simulink model "Lab1_Simulation"  (R2025b)
settings: Solver=VariableStepAuto  StartTime=0.0  StopTime=2  RelTol=1e-3
values from neighbouring files (symbols this model uses):
  a0 = K/a4    (= 224637.681159)    [Lab1matlab.m]
  a1 = (K*Tau1+K*Tau2+G)/a4    (= 24764.4927536)    [Lab1matlab.m]
  a2 = (Tau1*Tau2*K+G*Tau1+G*Tau2+J)/a4    (= 1527.89855072)    [Lab1matlab.m]
  a3 = (Tau1*Tau2*G+J*Tau1+J*Tau2)/a4    (= 60.8695652174)    [Lab1matlab.m]
  b0 = 1/a4    (= 226449.275362)    [Lab1matlab.m]
settings Model: Creator=peterbarkley  LastModifiedBy=peterbarkley

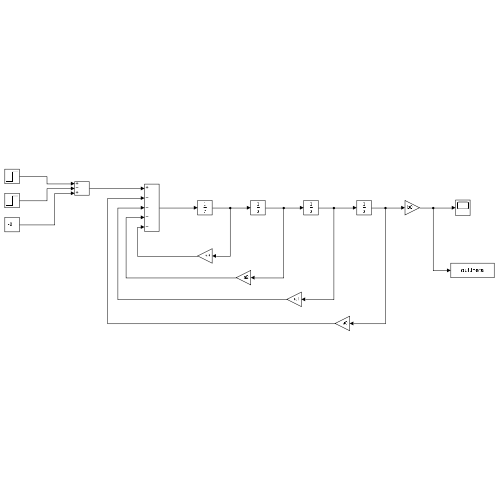
[thumbnail: Simulink's stored preview of the top-level diagram]
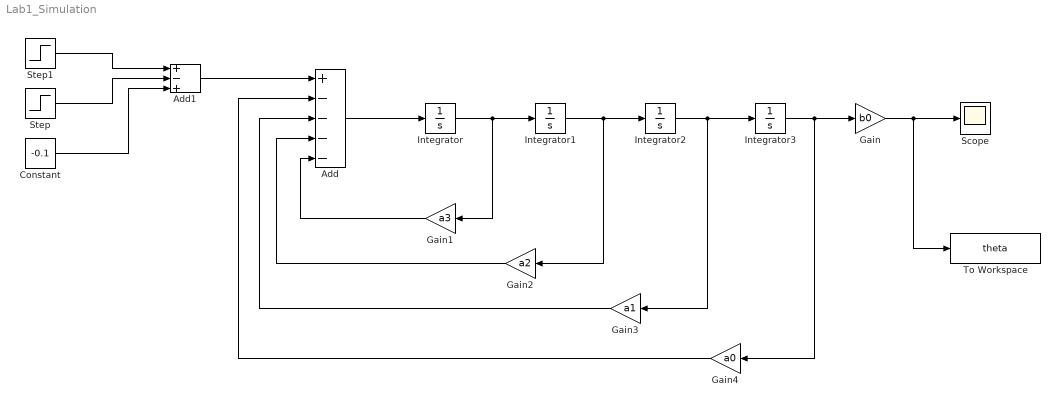
== system Lab1_Simulation ==
  Add : Sum  Inputs=+----
  Add1 : Sum  Inputs=+-+
  Constant : Constant  Value=-0.1
  Gain : Gain  Gain=b0
  Gain1 : Gain  Gain=a3
  Gain2 : Gain  Gain=a2
  Gain3 : Gain  Gain=a1
  Gain4 : Gain  Gain=a0
  Integrator{,1..3} (4 alike) : Integrator
  Scope : Scope
      settings: ActiveDisplayYMinimum=-0.38015343330105178  ActiveDisplayYMaximum=1.3949022843097443
  Step : Step  SampleTime=0
  Step1 : Step  Time=0  SampleTime=0
  To Workspace : ToWorkspace  VariableName=theta  SampleTime=-1
  wires:
  Add/1 -> Integrator/1
  Integrator/1 -> Gain1/1, Integrator1/1
  Gain1/1 -> Add/5
  Integrator1/1 -> Gain2/1, Integrator2/1
  Integrator2/1 -> Gain3/1, Integrator3/1
  Integrator3/1 -> Gain4/1, Gain/1
  Gain2/1 -> Add/4
  Gain3/1 -> Add/3
  Gain4/1 -> Add/2
  Gain/1 -> To Workspace/1, Scope/1
  Add1/1 -> Add/1
  Step/1 -> Add1/2
  Step1/1 -> Add1/1
  Constant/1 -> Add1/3
